simulink library "Thermostat_Proportional"  (R2018b)
settings: Solver=ode45  StartTime=0.0  StopTime=10.0  RelTol=1e-3  EnableMultiTasking=on
settings Model: Creator=lena.frank  LastModifiedBy=P41573
settings DataIOCC: LimitDataPoints=on  SaveFormat=Array  SignalLoggingSaveFormat=ModelDataLogs
settings OptimizationCC: ExpressionDepthLimit=2147483647  LifeSpan=inf
settings DebuggingCC: UnderspecifiedInitializationDetection=Classic  MergeDetectMultiDrivingBlocksExec=none  SolverPrmCheckMsg=warning  FcnCallInpInsideContextMsg=warning  StateNameClashWarn=warning  SFUnexpectedBacktrackingDiag=warning  SFNoUnconditionalDefaultTransitionDiag=warning  SFExecutionAtInitializationDiag=none
settings HardwareCC: ProdBitPerPointer=32  ProdBitPerSizeT=32  ProdBitPerPtrDiffT=32  ProdLargestAtomicFloat=None  ProdIntDivRoundTo=Undefined  ProdEndianess=Unspecified  ProdWordSize=32  ProdHWDeviceType=32-bit Generic
settings ModelReferenceCC: PropagateSignalLabelsOutOfModel=off
settings SFSimCC: SimUseLocalCustomCode=off
settings RTWCC: RTWUseLocalCustomCode=off
settings CodeAppCC: StateflowObjectComments=on
settings GRTTargetCC: TargetLangStandard=C89/C90 (ANSI)  GeneratePreprocessorConditionals=Disable all  CombineOutputUpdateFcns=off  GRTInterface=on
settings ConfigComp: CovMetricSettings=dw  CovHtmlReporting=on  CovSaveCumulativeToWorkspaceVar=on  CovSaveSingleToWorkspaceVar=on  CovExternalEMLEnable=off

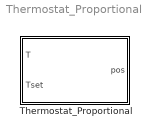
== system Thermostat_Proportional ==
  Thermostat_Proportional : Subsystem  mask(Thermostat){op=0.5, bl=0.2, p=4, ts=60}
      mask prompts: op "Operation point (valve position at set temperature)"; bl "Hysteresis or play in K"; p "Proportional range in K"; ts "First order hold for temperature sensor in s"
      mask help: Thermostat with proportional characteristic and play.
      mask TypeOptions op: operationPosition/Value
      mask TypeOptions bl: Play/Value | Backlash/BacklashWidth
      mask TypeOptions p: proportionalRange/Value
      mask TypeOptions ts: Sensor/ts
      mask Display: plot(-10,15,80,95,[10,20,30,40,40,30,20,10,10],[30,20,20,30,40,50,50,40,30],[40,60,60,50,40,30,10],[30,70,80,90,90,80,40],[50,30],[90,50],[60,40],[80,41],[40,20],[90,50],[19,11,14],[36,36,33],[23,26,29,29,25,28,23],[41,39,41,43,45,48,48],[32,31,32,35,35,38,38],[39,36,33,35,39,39,33])

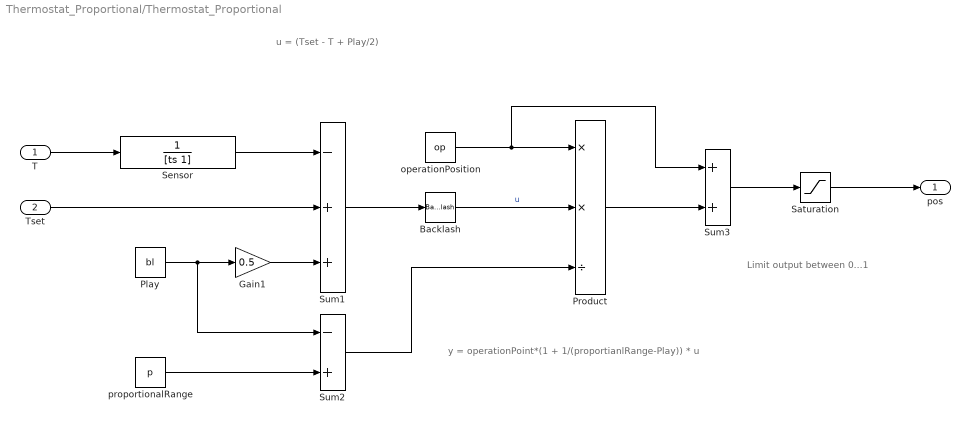
== system Thermostat_Proportional/Thermostat_Proportional ==
  note: Limit output between 0...1
  note: y = operationPoint*(1 + 1/(proportianlRange-Play)) * u
  note: u = (Tset - T + Play/2)
  T : Inport
  Tset : Inport  Port=2
  Backlash : Backlash  BacklashWidth=bl
  Gain1 : Gain  Gain=0.5
  Play : Constant  Value=bl
  Product : Product  Inputs=**/
  Saturation : Saturate  UpperLimit=1  LowerLimit=0
  Sensor : TransferFcn  Denominator=[ts 1]  mask{ts=ts}
      mask prompts: ts "First order hold for temperature sensor in s"
  Sum1 : Sum  Inputs=-++  SaturateOnIntegerOverflow=on  InputSameDT=on  OutDataTypeStr=Inherit: Same as first input
  Sum2 : Sum  Inputs=-+  SaturateOnIntegerOverflow=on  InputSameDT=on  OutDataTypeStr=Inherit: Same as first input
  Sum3 : Sum  Inputs=2  SaturateOnIntegerOverflow=on  InputSameDT=on  OutDataTypeStr=Inherit: Same as first input
  operationPosition : Constant  Value=op
  proportionalRange : Constant  Value=p
  pos : Outport
  wires:
  Product/1 -> Sum3/2
  Sum2/1 -> Product/3
  proportionalRange/1 -> Sum2/2
  operationPosition/1 -> Product/1, Sum3/1
  Gain1/1 -> Sum1/3
  Play/1 -> Gain1/1, Sum2/1
  Tset/1 -> Sum1/2
  T/1 -> Sensor/1
  Sum3/1 -> Saturation/1
  Saturation/1 -> pos/1
  Backlash/1 -> Product/2  "u"
  Sum1/1 -> Backlash/1
  Sensor/1 -> Sum1/1
